simulink model "sensor_model"  (R2018b)
settings: Solver=ode45  StartTime=0.0  StopTime=900  MaxStep=0.001  RelTol=1e-3
libraries: simulink x9
settings Model: Creator=LaAir  LastModifiedBy=LaAir

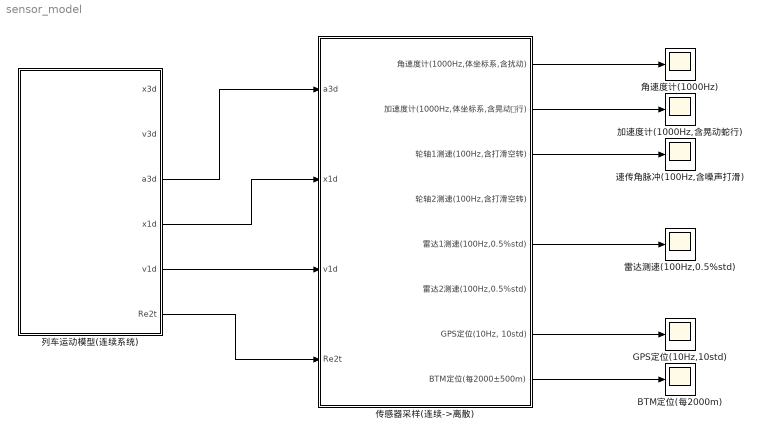
== system sensor_model ==
  BTM定位(每2000m) : Scope
  GPS定位(10Hz,10std) : Scope
  传感器采样(连续->离散) : Subsystem
  列车运动模型(连续系统) : Subsystem
  加速度计(1000Hz,含晃动蛇行) : Scope
  角速度计(1000Hz) : Scope
  速传角脉冲(100Hz,含噪声打滑) : Scope
  雷达测速(100Hz,0.5%std) : Scope
  wires:
  传感器采样(连续->离散)/2(加速度计(1000Hz,体坐标系,含晃动🐍行)) -> 加速度计(1000Hz,含晃动蛇行)/1
  传感器采样(连续->离散)/3(轮轴1测速(100Hz,含打滑空转)) -> 速传角脉冲(100Hz,含噪声打滑)/1
  传感器采样(连续->离散)/7("GPS定位(10Hz, 10std)") -> GPS定位(10Hz,10std)/1
  传感器采样(连续->离散)/8(BTM定位(每2000±500m)) -> BTM定位(每2000m)/1
  传感器采样(连续->离散)/5(雷达1测速(100Hz,0.5%std)) -> 雷达测速(100Hz,0.5%std)/1
  列车运动模型(连续系统)/4(x1d) -> 传感器采样(连续->离散)/2(x1d)
  列车运动模型(连续系统)/3(a3d) -> 传感器采样(连续->离散)/1(a3d)
  列车运动模型(连续系统)/5(v1d) -> 传感器采样(连续->离散)/3(v1d)
  列车运动模型(连续系统)/6(Re2t) -> 传感器采样(连续->离散)/4(Re2t)
  传感器采样(连续->离散)/1(角速度计(1000Hz,体坐标系,含扰动)) -> 角速度计(1000Hz)/1

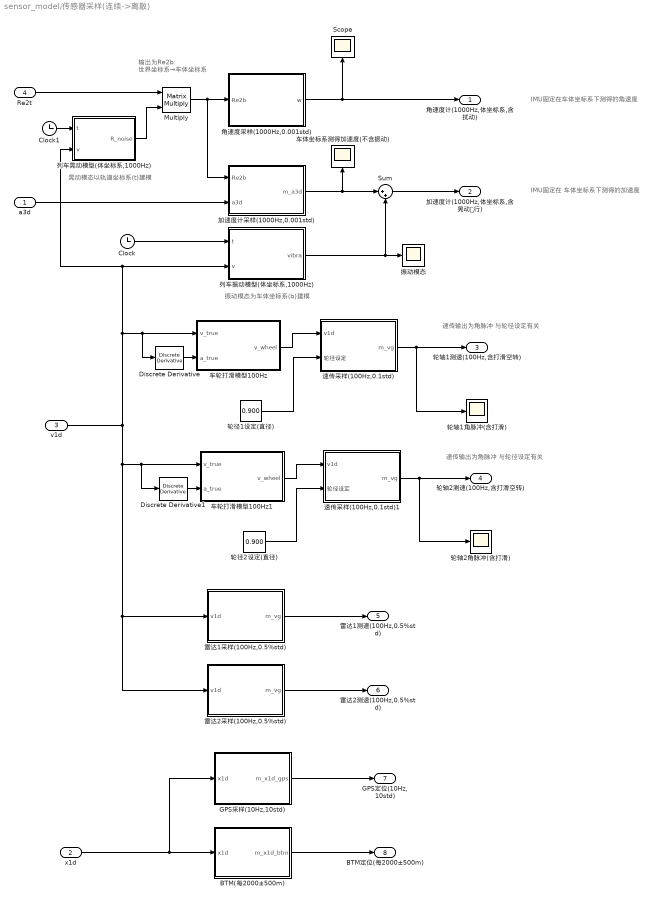
== system sensor_model/传感器采样(连续->离散) ==
  note: 速传输出为角脉冲
      | 与轮径设定有关
  note: 速传输出为角脉冲
      | 与轮径设定有关
  note: 输出为Re2b:
      | 世界坐标系→车体坐标系
  note: IMU固定在车体坐标系下测得的角速度
  note: IMU固定在 车体坐标系下测得的加速度
  note: 振动模态为车体坐标系(b)建模
  note: 晃动模态以轨道坐标系(t)建模
  a3d : Inport
  x1d : Inport  Port=2
  v1d : Inport  Port=3
  Re2t : Inport  Port=4
  BTM(每2000±500m) : Subsystem
  Clock : Clock
  Clock1 : Clock
  Discrete Derivative : simulink/Discrete/Discrete Derivative  gainval=1.0  ICPrevScaledInput=0.0  OutMin=[]  OutMax=[]  OutDataType=fixdt(1, 16)  OutScaling=2^-10  DoSatur=off
  Discrete Derivative1 : simulink/Discrete/Discrete Derivative  gainval=1.0  ICPrevScaledInput=0.0  OutMin=[]  OutMax=[]  OutDataType=fixdt(1, 16)  OutScaling=2^-10  DoSatur=off
  GPS采样(10Hz,10std) : Subsystem
  Multiply : Product  Multiplication=Matrix(*)
  Scope : Scope
  Sum : Sum  Inputs=|++
  列车振动模型(体坐标系,1000Hz) : MATLAB Function  TreatAsAtomicUnit=on  SystemSampleTime=1e-3
  列车晃动模型(体坐标系,1000Hz) : MATLAB Function  TreatAsAtomicUnit=on  SystemSampleTime=1e-3
  加速度计采样(1000Hz,0.001std) : Subsystem
  振动模态 : Scope
  角速度采样(1000Hz,0.001std) : Subsystem
  车体坐标系测得加速度(不含振动) : Scope
  车轮打滑模型100Hz : MATLAB Function  TreatAsAtomicUnit=on  SystemSampleTime=1e-2
  车轮打滑模型100Hz1 : MATLAB Function  TreatAsAtomicUnit=on  SystemSampleTime=1e-2
  轮径1设定(直径) : Constant  Value=0.900
  轮径2设定(直径) : Constant  Value=0.900
  轮轴1角脉冲(含打滑) : Scope
  轮轴2角脉冲(含打滑) : Scope
  速传采样(100Hz,0.1std) : Subsystem
  速传采样(100Hz,0.1std)1 : Subsystem
  雷达1采样(100Hz,0.5%std) : Subsystem
  雷达2采样(100Hz,0.5%std) : Subsystem
  角速度计(1000Hz,体坐标系,含扰动) : Outport
  加速度计(1000Hz,体坐标系,含晃动🐍行) : Outport  Port=2
  轮轴1测速(100Hz,含打滑空转) : Outport  Port=3
  轮轴2测速(100Hz,含打滑空转) : Outport  Port=4
  雷达1测速(100Hz,0.5%std) : Outport  Port=5
  雷达2测速(100Hz,0.5%std) : Outport  Port=6
  "GPS定位(10Hz, 10std)" : Outport  Port=7
  BTM定位(每2000±500m) : Outport  Port=8
  wires:
  x1d/1 -> GPS采样(10Hz,10std)/1(x1d), BTM(每2000±500m)/1(x1d)
  BTM(每2000±500m)/1(m_x1d_btm) -> BTM定位(每2000±500m)/1
  速传采样(100Hz,0.1std)/1(m_vg) -> 轮轴1角脉冲(含打滑)/1, 轮轴1测速(100Hz,含打滑空转)/1
  GPS采样(10Hz,10std)/1(m_x1d_gps) -> "GPS定位(10Hz, 10std)"/1
  a3d/1 -> 加速度计采样(1000Hz,0.001std)/2(a3d)
  轮径1设定(直径)/1 -> 速传采样(100Hz,0.1std)/2(轮径设定)
  雷达1采样(100Hz,0.5%std)/1(m_vg) -> 雷达1测速(100Hz,0.5%std)/1
  Discrete Derivative/1 -> 车轮打滑模型100Hz/2(a_true)
  车轮打滑模型100Hz/1(v_wheel) -> 速传采样(100Hz,0.1std)/1(v1d)
  Clock/1 -> 列车振动模型(体坐标系,1000Hz)/1(t)
  加速度计采样(1000Hz,0.001std)/1(m_a3d) -> 车体坐标系测得加速度(不含振动)/1, Sum/1
  Sum/1 -> 加速度计(1000Hz,体坐标系,含晃动🐍行)/1
  列车振动模型(体坐标系,1000Hz)/1(vibra) -> Sum/2, 振动模态/1
  车轮打滑模型100Hz1/1(v_wheel) -> 速传采样(100Hz,0.1std)1/1(v1d)
  轮径2设定(直径)/1 -> 速传采样(100Hz,0.1std)1/2(轮径设定)
  Discrete Derivative1/1 -> 车轮打滑模型100Hz1/2(a_true)
  速传采样(100Hz,0.1std)1/1(m_vg) -> 轮轴2角脉冲(含打滑)/1, 轮轴2测速(100Hz,含打滑空转)/1
  v1d/1 -> Discrete Derivative1/1, 车轮打滑模型100Hz1/1(v_true), 雷达2采样(100Hz,0.5%std)/1(v1d), 雷达1采样(100Hz,0.5%std)/1(v1d), 列车晃动模型(体坐标系,1000Hz)/2(v), 列车振动模型(体坐标系,1000Hz)/2(v), Discrete Derivative/1, 车轮打滑模型100Hz/1(v_true)
  雷达2采样(100Hz,0.5%std)/1(m_vg) -> 雷达2测速(100Hz,0.5%std)/1
  Re2t/1 -> Multiply/1
  列车晃动模型(体坐标系,1000Hz)/1(R_noise) -> Multiply/2
  Clock1/1 -> 列车晃动模型(体坐标系,1000Hz)/1(t)
  Multiply/1 -> 角速度采样(1000Hz,0.001std)/1(Re2b), 加速度计采样(1000Hz,0.001std)/1(Re2b)
  角速度采样(1000Hz,0.001std)/1(w) -> 角速度计(1000Hz,体坐标系,含扰动)/1, Scope/1

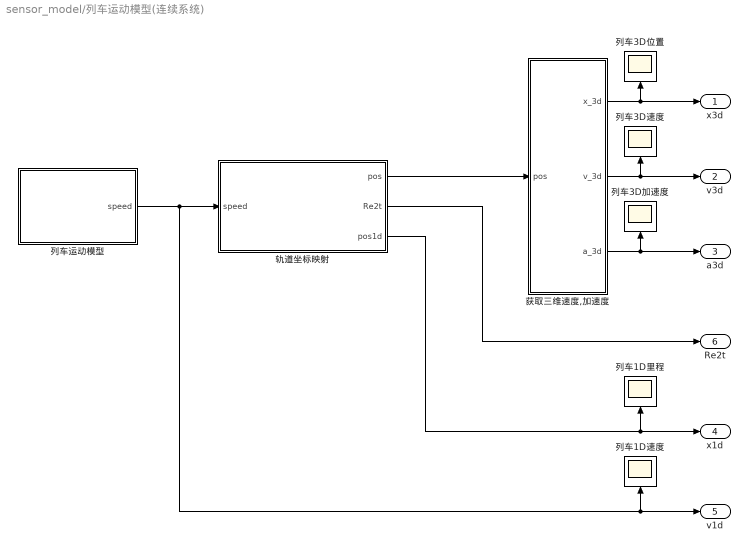
== system sensor_model/列车运动模型(连续系统) ==
  列车1D速度 : Scope
  列车1D里程 : Scope
  列车3D位置 : Scope
  列车3D加速度 : Scope
  列车3D速度 : Scope
  列车运动模型 : Subsystem
  获取三维速度,加速度 : Subsystem
  轨道坐标映射 : Subsystem
  x3d : Outport
  v3d : Outport  Port=2
  a3d : Outport  Port=3
  x1d : Outport  Port=4
  v1d : Outport  Port=5
  Re2t : Outport  Port=6
  wires:
  轨道坐标映射/1(pos) -> 获取三维速度,加速度/1(pos)
  获取三维速度,加速度/1(x_3d) -> 列车3D位置/1, x3d/1
  列车运动模型/1(speed) -> 轨道坐标映射/1(speed), 列车1D速度/1, v1d/1
  获取三维速度,加速度/3(a_3d) -> 列车3D加速度/1, a3d/1
  获取三维速度,加速度/2(v_3d) -> 列车3D速度/1, v3d/1
  轨道坐标映射/3(pos1d) -> x1d/1, 列车1D里程/1
  轨道坐标映射/2(Re2t) -> Re2t/1

== system sensor_model/传感器采样(连续->离散)/BTM(每2000±500m) ==
  note: BTM数据没有采样间隔，但是为了仿真同步，
      | 增加了最高采样速率作为基准频率
  x1d : Inport
  1000Hz : ZeroOrderHold  SampleTime=1e-3
  Constant : Constant  Value=2000
  MATLAB Function : MATLAB Function  TreatAsAtomicUnit=on
  m_x1d_btm : Outport
  wires:
  x1d/1 -> 1000Hz/1
  1000Hz/1 -> MATLAB Function/1(x1d)
  MATLAB Function/1(m_x1d_btm) -> m_x1d_btm/1
  Constant/1 -> MATLAB Function/2(gap)

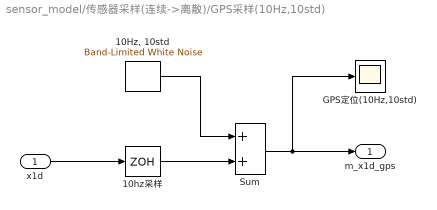
== system sensor_model/传感器采样(连续->离散)/GPS采样(10Hz,10std) ==
  x1d : Inport
  "10Hz, 10std" : simulink/Sources/Band-Limited White Noise  Cov=10  Ts=1e-1  seed=1006
  10hz采样 : ZeroOrderHold  SampleTime=1e-1
  GPS定位(10Hz,10std) : Scope
  Sum : Sum
  m_x1d_gps : Outport
  wires:
  x1d/1 -> 10hz采样/1
  "10Hz, 10std"/1 -> Sum/1
  10hz采样/1 -> Sum/2
  Sum/1 -> GPS定位(10Hz,10std)/1, m_x1d_gps/1

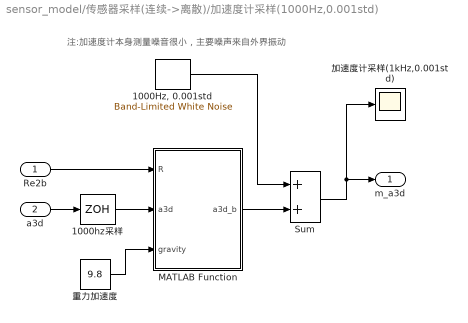
== system sensor_model/传感器采样(连续->离散)/加速度计采样(1000Hz,0.001std) ==
  note: 注:加速度计本身测量噪音很小，主要噪声来自外界振动
  Re2b : Inport
  a3d : Inport  Port=2
  "1000Hz, 0.001std" : simulink/Sources/Band-Limited White Noise  Cov=1e-9  Ts=1e-3  seed=1001
  1000hz采样 : ZeroOrderHold  SampleTime=1e-3
  MATLAB Function : MATLAB Function  TreatAsAtomicUnit=on
  Sum : Sum
  加速度计采样(1kHz,0.001std) : Scope
  重力加速度 : Constant  Value=9.8
  m_a3d : Outport
  wires:
  "1000Hz, 0.001std"/1 -> Sum/1
  MATLAB Function/1(a3d_b) -> Sum/2
  Sum/1 -> m_a3d/1, 加速度计采样(1kHz,0.001std)/1
  Re2b/1 -> MATLAB Function/1(R)
  a3d/1 -> 1000hz采样/1
  1000hz采样/1 -> MATLAB Function/2(a3d)
  重力加速度/1 -> MATLAB Function/3(gravity)

== system sensor_model/传感器采样(连续->离散)/角速度采样(1000Hz,0.001std) ==
  Re2b : Inport
  "1000Hz, 1e-3std" : simulink/Sources/Band-Limited White Noise  Cov=1e-9  Ts=1e-3  seed=1010
  Sum1 : Sum
  角速度采样(1000Hz) : MATLAB Function  TreatAsAtomicUnit=on  SystemSampleTime=1e-3
  w : Outport
  wires:
  "1000Hz, 1e-3std"/1 -> Sum1/1
  角速度采样(1000Hz)/1(w) -> Sum1/2
  Sum1/1 -> w/1
  Re2b/1 -> 角速度采样(1000Hz)/1(R)

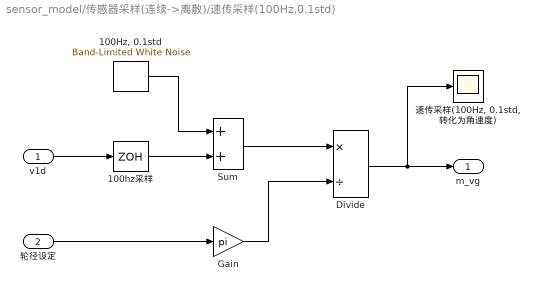
== system sensor_model/传感器采样(连续->离散)/速传采样(100Hz,0.1std) ==
  v1d : Inport
  轮径设定 : Inport  Port=2
  "100Hz, 0.1std" : simulink/Sources/Band-Limited White Noise  Cov=1e-4  Ts=1e-2  seed=1002
  100hz采样 : ZeroOrderHold  SampleTime=1e-2
  Divide : Product  Inputs=*/
  Gain : Gain  Gain=pi
  Sum : Sum
  "速传采样(100Hz, 0.1std, 转化为角速度)" : Scope
  m_vg : Outport
  wires:
  v1d/1 -> 100hz采样/1
  100hz采样/1 -> Sum/2
  Sum/1 -> Divide/1
  "100Hz, 0.1std"/1 -> Sum/1
  Divide/1 -> "速传采样(100Hz, 0.1std, 转化为角速度)"/1, m_vg/1
  Gain/1 -> Divide/2
  轮径设定/1 -> Gain/1

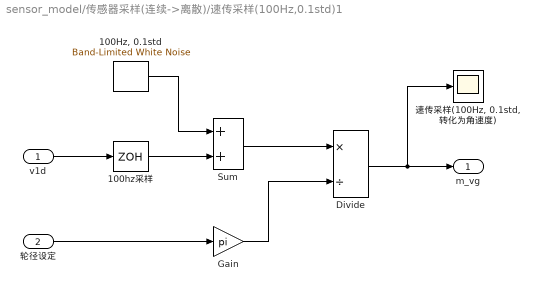
== system sensor_model/传感器采样(连续->离散)/速传采样(100Hz,0.1std)1 ==
  v1d : Inport
  轮径设定 : Inport  Port=2
  "100Hz, 0.1std" : simulink/Sources/Band-Limited White Noise  Cov=1e-4  Ts=1e-2  seed=1003
  100hz采样 : ZeroOrderHold  SampleTime=1e-2
  Divide : Product  Inputs=*/
  Gain : Gain  Gain=pi
  Sum : Sum
  "速传采样(100Hz, 0.1std, 转化为角速度)" : Scope
  m_vg : Outport
  wires:
  v1d/1 -> 100hz采样/1
  100hz采样/1 -> Sum/2
  Sum/1 -> Divide/1
  "100Hz, 0.1std"/1 -> Sum/1
  Divide/1 -> "速传采样(100Hz, 0.1std, 转化为角速度)"/1, m_vg/1
  Gain/1 -> Divide/2
  轮径设定/1 -> Gain/1

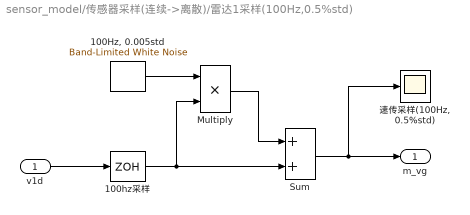
== system sensor_model/传感器采样(连续->离散)/雷达1采样(100Hz,0.5%std) ==
  v1d : Inport
  "100Hz, 0.005std" : simulink/Sources/Band-Limited White Noise  Cov=25e-8  Ts=1e-2  seed=1004
  100hz采样 : ZeroOrderHold  SampleTime=1e-2
  Multiply : Product
  Sum : Sum
  "速传采样(100Hz, 0.5%std)" : Scope
  m_vg : Outport
  wires:
  v1d/1 -> 100hz采样/1
  100hz采样/1 -> Multiply/2, Sum/2
  Sum/1 -> "速传采样(100Hz, 0.5%std)"/1, m_vg/1
  "100Hz, 0.005std"/1 -> Multiply/1
  Multiply/1 -> Sum/1

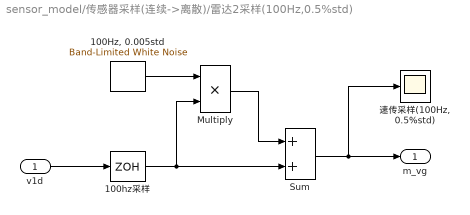
== system sensor_model/传感器采样(连续->离散)/雷达2采样(100Hz,0.5%std) ==
  v1d : Inport
  "100Hz, 0.005std" : simulink/Sources/Band-Limited White Noise  Cov=25e-8  Ts=1e-2  seed=1005
  100hz采样 : ZeroOrderHold  SampleTime=1e-2
  Multiply : Product
  Sum : Sum
  "速传采样(100Hz, 0.5%std)" : Scope
  m_vg : Outport
  wires:
  v1d/1 -> 100hz采样/1
  100hz采样/1 -> Multiply/2, Sum/2
  Sum/1 -> "速传采样(100Hz, 0.5%std)"/1, m_vg/1
  "100Hz, 0.005std"/1 -> Multiply/1
  Multiply/1 -> Sum/1

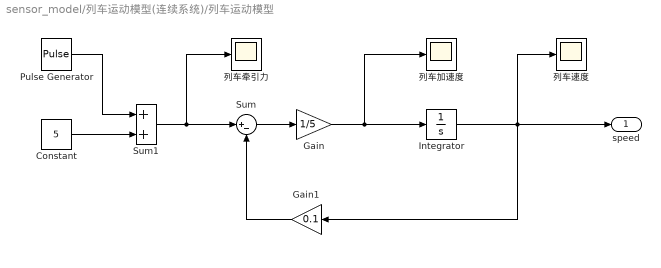
== system sensor_model/列车运动模型(连续系统)/列车运动模型 ==
  Constant : Constant  Value=5
  Gain : Gain  Gain=1/5
  Gain1 : Gain  Gain=0.1
  Integrator : Integrator
  Pulse Generator : DiscretePulseGenerator  PulseType=Time based  Amplitude=5  Period=600  PulseWidth=50
  Sum : Sum  Inputs=|+-
  Sum1 : Sum
  列车加速度 : Scope
  列车牵引力 : Scope
  列车速度 : Scope
  speed : Outport
  wires:
  Gain1/1 -> Sum/2
  Integrator/1 -> 列车速度/1, speed/1, Gain1/1
  Sum/1 -> Gain/1
  Gain/1 -> 列车加速度/1, Integrator/1
  Constant/1 -> Sum1/2
  Pulse Generator/1 -> Sum1/1
  Sum1/1 -> 列车牵引力/1, Sum/1

== system sensor_model/列车运动模型(连续系统)/获取三维速度,加速度 ==
  pos : Inport
  Derivative : Derivative
  Derivative1 : Derivative
  x_3d : Outport
  v_3d : Outport  Port=2
  a_3d : Outport  Port=3
  wires:
  Derivative/1 -> v_3d/1, Derivative1/1
  Derivative1/1 -> a_3d/1
  pos/1 -> x_3d/1, Derivative/1

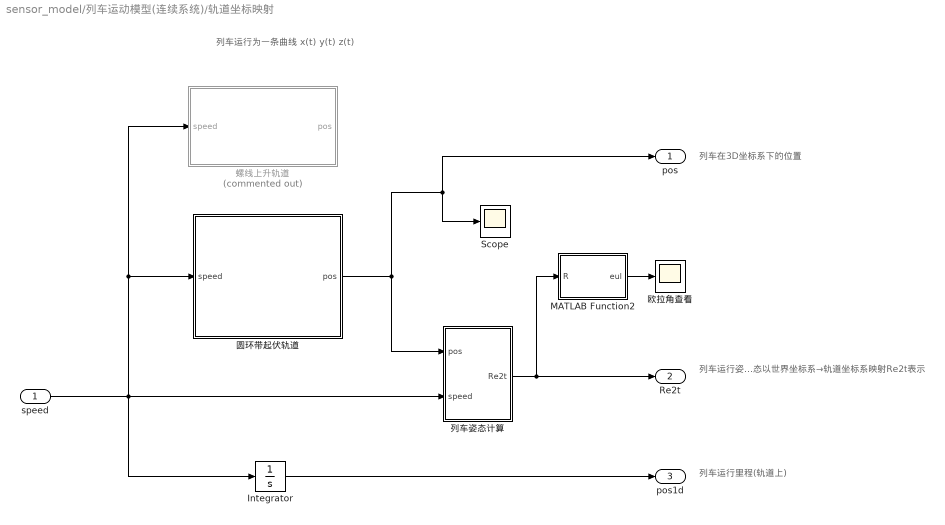
== system sensor_model/列车运动模型(连续系统)/轨道坐标映射 ==
  note: 列车运行为一条曲线
      | x(t) y(t) z(t)
  note: 列车运行里程(轨道上)
  note: 列车在3D坐标系下的位置
  note: 列车运行姿态以世界坐标系→轨道坐标系映射Re2t表示
  speed : Inport
  Integrator : Integrator
  MATLAB Function2 : MATLAB Function  TreatAsAtomicUnit=on
  Scope : Scope
  列车姿态计算 : Subsystem
  圆环带起伏轨道 : Subsystem
  欧拉角查看 : Scope
  螺线上升轨道 : Subsystem  Commented=on
  pos : Outport
  Re2t : Outport  Port=2
  pos1d : Outport  Port=3
  wires:
  speed/1 -> 螺线上升轨道/1(speed), 圆环带起伏轨道/1(speed), 列车姿态计算/2(speed), Integrator/1
  圆环带起伏轨道/1(pos) -> 列车姿态计算/1(pos), Scope/1, pos/1
  Integrator/1 -> pos1d/1
  列车姿态计算/1(Re2t) -> Re2t/1, MATLAB Function2/1(R)
  MATLAB Function2/1(eul) -> 欧拉角查看/1

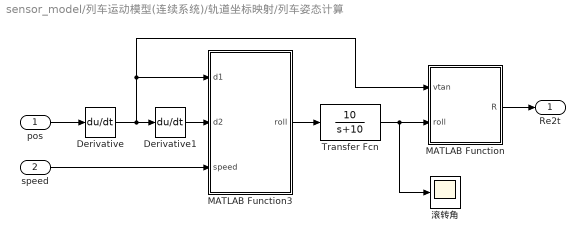
== system sensor_model/列车运动模型(连续系统)/轨道坐标映射/列车姿态计算 ==
  pos : Inport
  speed : Inport  Port=2
  Derivative : Derivative  CoefficientInTFapproximation=100
  Derivative1 : Derivative  CoefficientInTFapproximation=100
  MATLAB Function : MATLAB Function  TreatAsAtomicUnit=on
  MATLAB Function3 : MATLAB Function  TreatAsAtomicUnit=on
  Transfer Fcn : TransferFcn  Numerator=[10]  Denominator=[1 10]
  滚转角 : Scope
  Re2t : Outport
  wires:
  MATLAB Function/1(R) -> Re2t/1
  Derivative1/1 -> MATLAB Function3/2(d2)
  pos/1 -> Derivative/1
  Derivative/1 -> MATLAB Function3/1(d1), MATLAB Function/1(vtan), Derivative1/1
  Transfer Fcn/1 -> 滚转角/1, MATLAB Function/2(roll)
  speed/1 -> MATLAB Function3/3(speed)
  MATLAB Function3/1(roll) -> Transfer Fcn/1

== system sensor_model/列车运动模型(连续系统)/轨道坐标映射/圆环带起伏轨道 ==
  note: z(s)=Asin(Lz​2π​s+φ)
      | g(s)=dsdz​=A(Lz​2π​)cos(Lz​2π​s+φ)
  speed : Inport
  Integrator1 : Integrator
  Integrator2 : Integrator
  MATLAB Function1 : MATLAB Function  TreatAsAtomicUnit=on
  pos : Outport
  wires:
  speed/1 -> MATLAB Function1/2(v), Integrator2/1
  Integrator1/1 -> MATLAB Function1/3(theta)
  Integrator2/1 -> MATLAB Function1/1(s)
  MATLAB Function1/1(theta_dot) -> Integrator1/1
  MATLAB Function1/2(pos) -> pos/1

== system sensor_model/列车运动模型(连续系统)/轨道坐标映射/螺线上升轨道 ==
  speed : Inport
  Integrator : Integrator
  MATLAB Function : MATLAB Function  TreatAsAtomicUnit=on
  pos : Outport
  wires:
  MATLAB Function/1(pos) -> pos/1
  Integrator/1 -> MATLAB Function/1(s)
  speed/1 -> Integrator/1

== matlab function sensor_model/列车运动模型(连续系统)/轨道坐标映射/圆环带起伏轨道/MATLAB Function1 ==
  data: theta_dot output; s input; pos output; v input; theta input
function [theta_dot, pos] = circleUndulate(s, v, theta)
% s    : 弧长（外部由 v 积分得到）
% v    : 速度
% R    : 半径
R = 10000;
% A,Lz,phi: 起伏参数；Lz列车行进多少米完成一次起伏
A = 20; Lz = 5000; phi = 0;
% theta: 当前角
% z0   : 初始高程基准
z0 = 0;
% 输出:
%   theta_dot = dθ/dt (供外部 Integrator)
%   z_dot     = dz/dt (供外部 Integrator, 可选)
%   x,y,z     = 当前位置

omega = 2*pi / Lz;
z_rel = A * sin(omega*s + phi);                % 相对起伏
g = A * omega * cos(omega*s + phi);            % dz/ds
if abs(g) >= 1
    g = 0.999999 * sign(g);
end

omega_s = sqrt(1 - g*g) / R;                   % dθ/ds
theta_dot = omega_s * v;                       % dθ/dt
% z_dot     = g * v;                             % dz/dt (如果想对 z 再积分)
x = R * cos(theta);
y = R * sin(theta);
z = z0 + z_rel;
pos = [x,y,z];
end

== matlab function sensor_model/列车运动模型(连续系统)/轨道坐标映射/螺线上升轨道/MATLAB Function ==
  data: s input; pos output
function pos = mapHelix_byGrade(s)
% s     : 沿轨道弧长（由积分器得到）
% R     : 半径 (m)
R = 10000;
% g     : 坡度 = dz/ds（如 2% 取 0.02）
g = 0.02;
% theta0: 初始角 (rad)
theta0 = 0;
% z0    : 初始高度 (m)
z0 = 0;

% 数值保护，避免 |g|>=1
if abs(g) >= 1
    if g >= 0
        g = 1 - 1e-9;
    else
        g = -1 + 1e-9;
    end
end

omega = sqrt(1 - g*g) / R;      % dθ/ds
theta = theta0 + omega .* s;

x = R .* cos(theta);
y = R .* sin(theta);
z = z0 + g .* s;
pos = [x,y,z];
end

== matlab function sensor_model/传感器采样(连续->离散)/BTM(每2000±500m)/MATLAB Function ==
  data: x1d input; m_x1d_btm output; gap input; jitter input
function m_x1d_btm = BTM(x1d, gap, jitter)
    % gap     : 基础间隔（比如 2000）
    % jitter  : 允许的随机扰动范围（比如 500）

    % 为本次计算生成一个随机间隔
    rand_gap = gap + (2*rand-1) * jitter;   % gap ± jitter

    % 按这个随机间隔向下取整
    m_x1d_btm = floor(x1d / rand_gap) * rand_gap;
end

== matlab function sensor_model/传感器采样(连续->离散)/车轮打滑模型100Hz ==
  data: v_true input; v_wheel output; a_true input
function v_wheel = fcn(v_true, a_true)
% v_true : 真实速度
% a_true : 真实加速度 (m/s^2)
% slip_max : 最大滑移率 (e.g. 0.05)
slip_max = 0.05;
% prob : 在加速/制动时发生打滑的概率 (0~1),需要除以采样间隔代表每秒触发率
prob = 0.05/100;  % 100Hz

persistent isSlip slip_sign slip_val
persistent init
if isempty(init)
    rng('shuffle');
    init = true;
end

if isempty(isSlip)
    isSlip = false;
    slip_sign = 0;
    slip_val = 0;
end

% 判断是否触发新一次打滑/空转
if ~isSlip && rand < prob * abs(a_true)
    % 开始一次事件
    isSlip = true;
    slip_sign = sign(a_true);      % +1=空转, -1=打滑
    slip_val = slip_max * rand;    % 随机强度
end

% 模拟持续若干秒（可加一个持续时间计数器）
if isSlip
    v_wheel = v_true * (1 + slip_sign*slip_val);
    % 简单起见，这里在速度下降/上升时结束事件
    if rand < 0.01
        isSlip = false;
    end
else
    v_wheel = v_true;
end

== matlab function sensor_model/传感器采样(连续->离散)/列车振动模型(体坐标系,1000Hz) ==
  data: t input; vibra output; v input
function vibra = vibration(t, v)
% 三维振动干扰 (速度依赖)
% 输入:
%   t - 仿真时间 (s)
%   v - 列车速度 (m/s)
% 输出:
%   ax, ay, az - 三个方向的加速度干扰 (m/s^2)

g = 9.81;  % 重力加速度

% ========== X 方向 (纵向) ==========
% 低频 (纵向起伏)
f_x_low = 0.5 + 0.002*v;
amp_x_low = (0.02 + 0.0002*v) * g;
x_low = amp_x_low * sin(2*pi*f_x_low*t);

% 高频 (轮轨冲击)
D = 0.92;   % 轮径 (m)
f_x_high = v / (pi*D);  % 轮对激励频率
amp_x_high = 0.01 * g;
x_high = amp_x_high * sin(2*pi*f_x_high*t);

ax = x_low + x_high;

% ========== Y 方向 (横向) ==========
% 蛇行运动 (速度依赖)
f_y_hunt = 0.3 + 0.004*v;
amp_y_hunt = (0.05 + 0.0005*v) * g;
y_hunt = amp_y_hunt * sin(2*pi*f_y_hunt*t);

% 中频横向不平顺
f_y_mid = v / 80;   % 对应轨道波长 ~80m
amp_y_mid = 0.02 * g;
y_mid = amp_y_mid * sin(2*pi*f_y_mid*t);

ay = y_hunt + y_mid;

% ========== Z 方向 (垂向) ==========
% 中频垂向振动
f_z_mid = v / 40;   % 对应轨道波长 ~40m
amp_z_mid = (0.05 + 0.0003*v) * g;
z_mid = amp_z_mid * sin(2*pi*f_z_mid*t);

% 瞬态冲击 (道岔/隧道)
pulse_interval = 100;  % 每x秒一次
pulse_width    = 0.3; % 持续0.3秒
if mod(t, pulse_interval) < pulse_width
    z_pulse = 0.1 * g + 0.0005*v;
else
    z_pulse = 0;
end

az = z_mid + z_pulse;
% az = z_mid;
vibra = [ax, ay, az];
end

== matlab function sensor_model/传感器采样(连续->离散)/角速度采样(1000Hz,0.001std)/角速度采样(1000Hz) ==
  data: R input; w output
function w = fcn(R)
dt = 1e-3;
persistent R_pre;
if isempty(R_pre)
    R_pre = R;
end

dR = (R - R_pre) / dt;
R_pre = R;
Omega = R' * dR;
w = [Omega(3,2); Omega(1,3); Omega(2,1)];

== matlab function sensor_model/传感器采样(连续->离散)/车轮打滑模型100Hz1 ==
  data: v_true input; v_wheel output; a_true input
function v_wheel = fcn(v_true, a_true)
% v_true : 真实速度
% a_true : 真实加速度 (m/s^2)
% slip_max : 最大滑移率 (e.g. 0.05)
slip_max = 0.05;
% prob : 在加速/制动时发生打滑的概率 (0~1),需要除以采样间隔代表每秒触发率
prob = 0.05/100;  % 100Hz

persistent isSlip slip_sign slip_val
persistent init
if isempty(init)
    rng('shuffle');
    init = true;
end

if isempty(isSlip)
    isSlip = false;
    slip_sign = 0;
    slip_val = 0;
end

% 判断是否触发新一次打滑/空转
if ~isSlip && rand < prob * abs(a_true)
    % 开始一次事件
    isSlip = true;
    slip_sign = sign(a_true);      % +1=空转, -1=打滑
    slip_val = slip_max * rand;    % 随机强度
end

% 模拟持续若干秒（可加一个持续时间计数器）
if isSlip
    v_wheel = v_true * (1 + slip_sign*slip_val);
    % 简单起见，这里在速度下降/上升时结束事件
    if rand < 0.01
        isSlip = false;
    end
else
    v_wheel = v_true;
end

== matlab function sensor_model/传感器采样(连续->离散)/列车晃动模型(体坐标系,1000Hz) ==
  data: t input; R_noise output; v input
function R_noise = fcn(t, v)
% t: 时间(s)   v: 速度(m/s)
% 输出: R_noise (局部->局部有扰动)

    % ----- 相位状态（保证连续） -----
    persistent phi_r phi_p phi_y last_t
    if isempty(last_t)
        phi_r = 0; phi_p = 0; phi_y = 0; last_t = t;
    end
    dt = max(t - last_t, 1e-6);   % 防止0步长
    last_t = t;

    % ----- 速度相关的“幅值 & 频率”模型（可按实测调整/限幅） -----
    % roll（横摇）：频率近似固定，幅值随速增大
    A_roll = deg2rad(0.5 + 0.005*v);                    % rad
    A_roll = min(A_roll, deg2rad(3));                   % 合理上限
    f_roll = 0.8;                                       % Hz

    % pitch（俯仰）：频率近似固定，幅值随速增大
    A_pitch = deg2rad(0.3 + 0.003*v);
    A_pitch = min(A_pitch, deg2rad(1.5));
    f_pitch = 1.5;                                      % Hz

    % yaw（蛇行）：频率随速增加，幅值随速增加
    Lc = 10;                                            % m，特征蛇行波长
    f_yaw = v / (2*pi*Lc);                              % Hz ≈ v/(2πLc)
    f_yaw = min(max(f_yaw, 0.3), 6.0);                  % 合理范围
    A_yaw = deg2rad(0.2 + 0.004*v);
    A_yaw = min(A_yaw, deg2rad(2));

    % ----- 积分频率得到相位（保证连续） -----
    phi_r = wrapPi(phi_r + 2*pi*f_roll*dt);
    phi_p = wrapPi(phi_p + 2*pi*f_pitch*dt);
    phi_y = wrapPi(phi_y + 2*pi*f_yaw*dt);

    % ----- 角度扰动（小角度，单位 rad） -----
    droll  = A_roll  * sin(phi_r);
    dpitch = A_pitch * sin(phi_p);
    dyaw   = A_yaw   * sin(phi_y);

    % ----- ZYX 欧拉 -> 旋转矩阵 -----
    cz = cos(dyaw);  sz = sin(dyaw);
    cy = cos(dpitch); sy = sin(dpitch);
    cx = cos(droll);  sx = sin(droll);

    Rz = [cz -sz 0; sz cz 0; 0 0 1];
    Ry = [cy 0 sy; 0 1 0; -sy 0 cy];
    Rx = [1 0 0; 0 cx -sx; 0 sx cx];

    R_noise = Rz * Ry * Rx;
end

function a = wrapPi(a)
% 把角度包到 [-pi, pi]
    a = mod(a + pi, 2*pi) - pi;
end

== matlab function sensor_model/传感器采样(连续->离散)/加速度计采样(1000Hz,0.001std)/MATLAB Function ==
  data: R input; a3d_b output; a3d input; gravity input
function a3d_b = fcn(R, a3d, gravity)
a3d(3) = a3d(3)-gravity;
y = R'*a3d';
a3d_b = y';

== matlab function sensor_model/列车运动模型(连续系统)/轨道坐标映射/列车姿态计算/MATLAB Function ==
  data: vtan input; R output; roll input
function R = fcn(vtan, roll)
% --- 轨道姿态 ---
x_axis = vtan / norm(vtan);            % 切向量 = 局部 x 轴
z_world = [0 0 1];           % 世界竖直方向

% Gram–Schmidt 正交化，得到局部 z 轴
z_axis = z_world - dot(z_world, x_axis)*x_axis;
z_axis = z_axis / norm(z_axis);

% y 轴由右手定则确定
y_axis = cross(z_axis, x_axis);
y_axis = y_axis / norm(y_axis);

% 以切向量 x_axis 为旋转轴，绕 roll 旋转
K = [ 0  0  0;
      0  0 -1;
      0  1  0 ];
R_roll = eye(3) + sin(roll)*K + (1-cos(roll))*(K*K);

% 世界->轨道 旋转矩阵 (列向量为局部基)
R = [x_axis(:), y_axis(:), z_axis(:)] * R_roll;

== matlab function sensor_model/列车运动模型(连续系统)/轨道坐标映射/列车姿态计算/MATLAB Function3 ==
  data: d1 input; roll output; d2 input; speed input
function roll = fcn(d1, d2, speed)
r = norm(d1(1:2))^3/norm(d1(1)*d2(2)-d1(2)*d2(1));
g = 9.8;
a = speed^2/r;
a = min(4, a);
roll = atan(a/g);

== matlab function sensor_model/列车运动模型(连续系统)/轨道坐标映射/MATLAB Function2 ==
  data: R input; eul output
 function eul = deg(R)
[U, ~, V] = svd(R);
R = U * V';
yaw = atan2(R(2,1),R(1,1));
pitch = asin(-R(3,1));
roll = atan2(R(3,2),R(3,3));
eul = [yaw, pitch, roll]*180/pi;
